simulink model "flightControlSystem"  (R2024b)
settings: Solver=ode3  StartTime=0  StopTime=TFinal  FixedStep=Ts  RelTol=1e-3  EnableMultiTasking=on
undefined symbols (not defined in the file): Ts, Vehicle
libraries: simulink x1
settings Model: ExtModeTrigDuration=80  Creator=The MathWorks, Inc.  LastModifiedBy=jadwe
settings SolverCC: AlgebraicLoopSolver=TrustRegion
settings DataIOCC: LimitDataPoints=on  SaveFormat=StructureWithTime  ReturnWorkspaceOutputs=off
settings OptimizationCC: BlockReduction=off  EnhancedBackFolding=on  PassReuseOutputArgsThreshold=0  MaxStackSize=64  OptimizeBlockOrder=speed  DifferentSizesBufferReuse=on  OptimizationCustomize=off
settings DebuggingCC: AlgebraicLoopMsg=none  ParameterPrecisionLossMsg=none  ParameterTunabilityLossMsg=error  BusObjectLabelMismatch=error  PregeneratedLibrarySubsystemCodeDiagnostic=none  SFUnexpectedBacktrackingDiag=warning  SFNoUnconditionalDefaultTransitionDiag=warning  SFExecutionAtInitializationDiag=none  ArithmeticOperatorsInVariantConditions=warning
settings HardwareCC: ProdBitPerPointer=32  ProdBitPerSizeT=32  ProdBitPerPtrDiffT=32  ProdLargestAtomicInteger=Long  ProdWordSize=32  ProdHWDeviceType=ARM Compatible->ARM 9  UseEmbeddedCoderFeatures=off  UseSimulinkCoderFeatures=off
settings ModelReferenceCC: EnableRefExpFcnMdlSchedulingChecks=on  ModelReferenceNumInstancesAllowed=Single  PropagateSignalLabelsOutOfModel=off
settings SFSimCC: SimUseLocalCustomCode=off  MATLABDynamicMemAlloc=off
settings RTWCC: Description=Embedded Coder  SystemTargetFile=ert.tlc  TemplateMakefile=ert_default_tmf  RTWUseLocalCustomCode=off  GPUComputeCapability=3.5  DLArmComputeVersion=19.05
settings CodeAppCC: ForceParamTrailComments=on  MaxIdLength=63  OperatorAnnotations=on
settings ERTTargetCC: ERTCustomFileBanners=off  MatFileLogging=on  SupportContinuousTime=on  SupportNonInlinedSFcns=on  RemoveResetFunc=off  ModelStepFunctionPrototypeControlCompliant=off  InlinedParameterPlacement=Hierarchical  ERTCustomFileTemplate=example_file_process.tlc  DynamicArrayContainerType=coder::array
settings ConfigComp: CovMetricSettings=dw  CovSaveCumulativeToWorkspaceVar=on  CovSaveSingleToWorkspaceVar=on  CovExternalEMLEnable=off  CovSFcnEnable=off

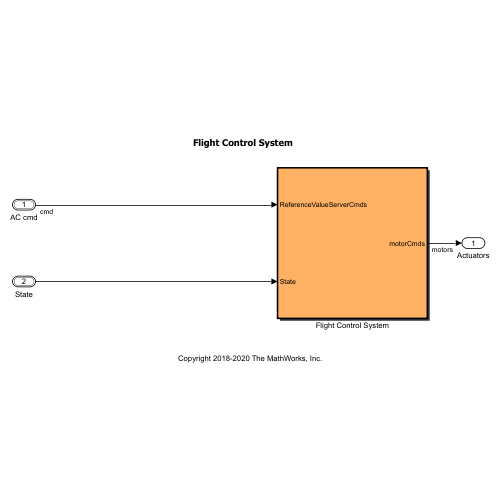
[thumbnail: Simulink's stored preview of the top-level diagram]
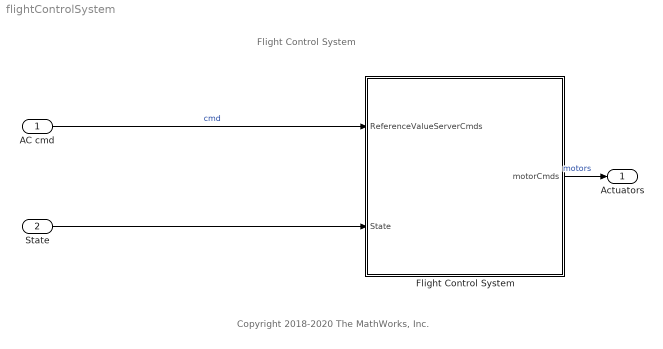
== system flightControlSystem ==
  note: Copyright 2018-2020 The MathWorks, Inc.
  note: Flight Control System
  AC cmd : Inport  OutDataTypeStr=Bus: CommandBus  BusOutputAsStruct=on
  State : Inport  Port=2  OutDataTypeStr=Bus: StateVectBus
  Flight Control System : Subsystem  TreatAsAtomicUnit=on  SystemSampleTime=Ts
  Actuators : Outport  OutDataTypeStr=single  PortDimensions=4  VectorParamsAs1DForOutWhenUnconnected=off
  wires:
  AC cmd/1 -> Flight Control System/1(ReferenceValueServerCmds)  "cmd"
  Flight Control System/1(motorCmds) -> Actuators/1  "motors"
  State/1 -> Flight Control System/2(State)

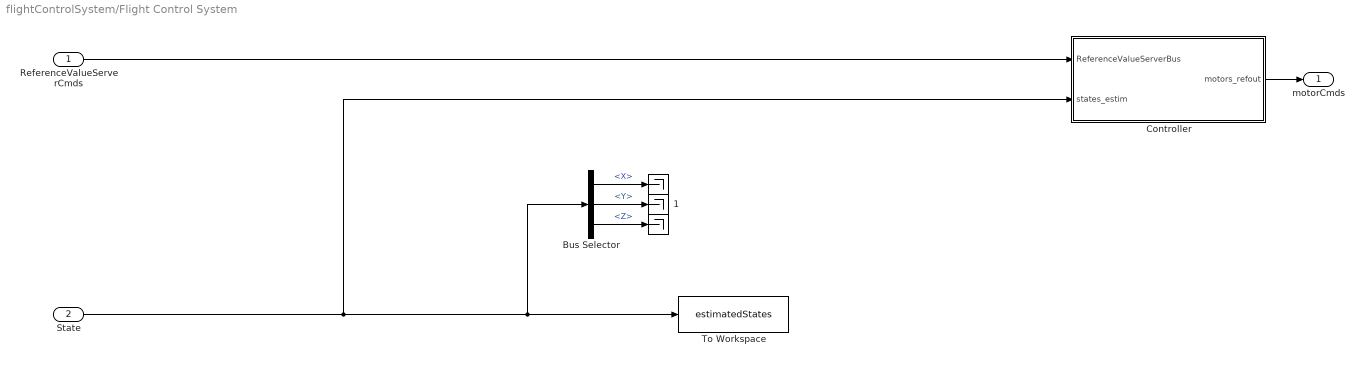
== system flightControlSystem/Flight Control System ==
  ReferenceValueServerCmds : Inport  OutDataTypeStr=Bus: CommandBus
  State : Inport  Port=2  OutDataTypeStr=Bus: StateVectBus
  " " : Terminator
  "    " : Terminator
  " 1" : Terminator
  Bus Selector : BusSelector  OutputSignals=X,Y,Z
  Controller : Subsystem
  To Workspace : ToWorkspace  VariableName=estimatedStates  SaveFormat=Structure With Time  SampleTime=-1
  motorCmds : Outport  VectorParamsAs1DForOutWhenUnconnected=off
  wires:
  State/1 -> Controller/2(states_estim), Bus Selector/1, To Workspace/1
  Bus Selector/1 -> " "/1  "<X>"
  Bus Selector/3 -> "    "/1  "<Z>"
  Bus Selector/2 -> " 1"/1  "<Y>"
  ReferenceValueServerCmds/1 -> Controller/1(ReferenceValueServerBus)
  Controller/1(motors_refout) -> motorCmds/1

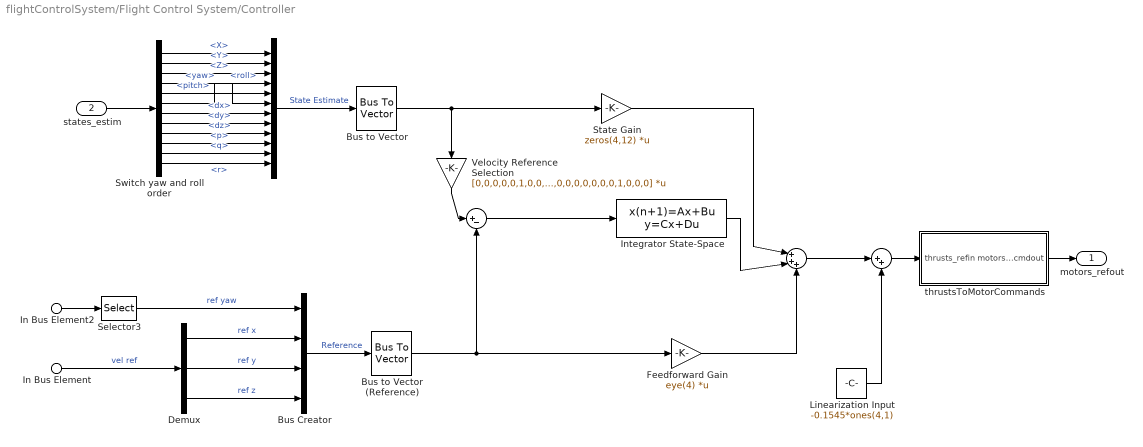
== system flightControlSystem/Flight Control System/Controller ==
  In Bus Element : Inport  PortName=ReferenceValueServerBus  Element=pos_ref
  In Bus Element2 : Inport  PortName=ReferenceValueServerBus  Element=orient_ref
  states_estim : Inport  Port=2
  " " : Sum  Inputs=|++
  "  " : Sum  Inputs=|+-
  "   " : BusCreator  Inputs=12
  "     " : Sum  Inputs=|+++
  Bus Creator : BusCreator  Inputs=4
  Bus to Vector : BusToVector
  Bus to Vector (Reference) : BusToVector
  Demux : Demux  Outputs=3
  Feedforward Gain : Gain  Gain=eye(4)  Multiplication=Matrix(K*u)
  Integrator State-Space : DiscreteStateSpace  A=0  B=zeros(1,4)  C=0  D=-zeros(1,4)  SampleTime=-1
  Linearization Input : Constant  Value=-0.1545*ones(4,1)  OutDataTypeStr=single
  Selector3 : Selector  InputPortWidth=3  IndexOptions=Index vector (dialog)  Indices=1  OutputSizes=1
  State Gain : Gain  Gain=zeros(4,12)  Multiplication=Matrix(K*u)
  Switch yaw and roll order : BusSelector  OutputSignals=X,Y,Z,yaw,pitch,roll,dx,dy,dz,p,q,r
  Velocity Reference Selection : Gain  Gain=[0,0,0,0,0,1,0,0,0,0,0,0;0,0,0,0,0,0,1,0,0,0,0,0;0,0,0,0,0,0,0,1,0,0,0,0;0,0,0,0,0,0,0,0,1,0,0,0]  Multiplication=Matrix(K*u)
  thrustsToMotorCommands : Subsystem
  motors_refout : Outport  VectorParamsAs1DForOutWhenUnconnected=off
  wires:
  Integrator State-Space/1 -> "     "/2
  Switch yaw and roll order/2 -> "   "/2  "<Y>"
  Selector3/1 -> Bus Creator/1  "ref yaw"
  Bus Creator/1 -> Bus to Vector (Reference)/1  "Reference"
  Demux/3 -> Bus Creator/4  "ref z"
  State Gain/1 -> "     "/1
  Velocity Reference Selection/1 -> "  "/1
  Switch yaw and roll order/8 -> "   "/8  "<dy>"
  states_estim/1 -> Switch yaw and roll order/1
  Bus to Vector/1 -> Velocity Reference Selection/1, State Gain/1
  "  "/1 -> Integrator State-Space/1
  Switch yaw and roll order/1 -> "   "/1  "<X>"
  Switch yaw and roll order/7 -> "   "/7  "<dx>"
  " "/1 -> thrustsToMotorCommands/1(thrusts_refin)
  Switch yaw and roll order/4 -> "   "/6  "<yaw>"
  Feedforward Gain/1 -> "     "/3
  Switch yaw and roll order/12 -> "   "/12  "<r>"
  "     "/1 -> " "/1
  Switch yaw and roll order/10 -> "   "/10  "<p>"
  Switch yaw and roll order/6 -> "   "/4  "<roll>"
  Switch yaw and roll order/11 -> "   "/11  "<q>"
  In Bus Element2/1 -> Selector3/1
  "   "/1 -> Bus to Vector/1  "State Estimate"
  Demux/1 -> Bus Creator/2  "ref x"
  Switch yaw and roll order/9 -> "   "/9  "<dz>"
  Switch yaw and roll order/3 -> "   "/3  "<Z>"
  In Bus Element/1 -> Demux/1  "vel ref"
  Bus to Vector (Reference)/1 -> Feedforward Gain/1, "  "/2
  thrustsToMotorCommands/1(motors_cmdout) -> motors_refout/1
  Switch yaw and roll order/5 -> "   "/5  "<pitch>"
  Demux/2 -> Bus Creator/3  "ref y"
  Linearization Input/1 -> " "/2

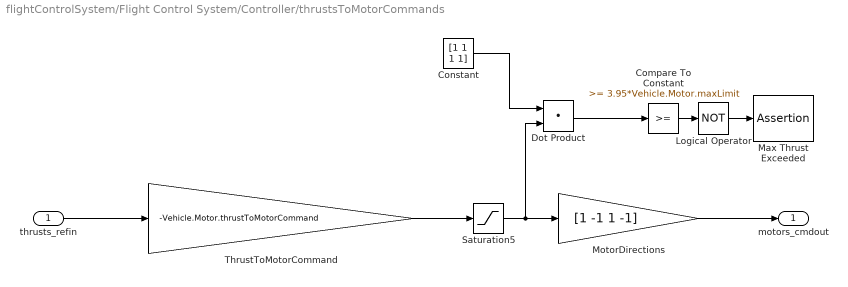
== system flightControlSystem/Flight Control System/Controller/thrustsToMotorCommands ==
  thrusts_refin : Inport
  Compare To Constant : simulink/Logic and Bit Operations/Compare To Constant  relop=>=  const=3.95*Vehicle.Motor.maxLimit  OutDataTypeStr=boolean
  Constant : Constant  Value=[1 1 1 1]  OutDataTypeStr=single
  Dot Product : DotProduct  OutDataTypeStr=Inherit: Inherit via internal rule
  Logical Operator : Logic  Operator=NOT  AllPortsSameDT=off  OutDataTypeStr=boolean
  Max Thrust Exceeded : Assertion
  MotorDirections : Gain  Gain=[1 -1 1 -1]
  Saturation5 : Saturate  UpperLimit=Vehicle.Motor.maxLimit  LowerLimit=Vehicle.Motor.minLimit
  ThrustToMotorCommand : Gain  Gain=-Vehicle.Motor.thrustToMotorCommand
  motors_cmdout : Outport  VectorParamsAs1DForOutWhenUnconnected=off
  wires:
  ThrustToMotorCommand/1 -> Saturation5/1
  thrusts_refin/1 -> ThrustToMotorCommand/1
  MotorDirections/1 -> motors_cmdout/1
  Dot Product/1 -> Compare To Constant/1
  Compare To Constant/1 -> Logical Operator/1
  Saturation5/1 -> Dot Product/2, MotorDirections/1
  Logical Operator/1 -> Max Thrust Exceeded/1
  Constant/1 -> Dot Product/1
